simulink model "fir_fft"  (R2022a)
settings: Solver=VariableStepAuto  StartTime=0.0  StopTime=1024*inf  RelTol=1e-3
undefined symbols (not defined in the file): S, taps_td, vsva2197, xcvc1902
libraries: aieBasic x5, aieDSP x2, dspsrcs4 x1, vmcUtilities x1
settings Model: Creator=abehbood  LastModifiedBy=abehbood
settings ModelReferenceCC: EnableRefExpFcnMdlSchedulingChecks=off
settings RTWCC: Description=Generic Real-Time Target

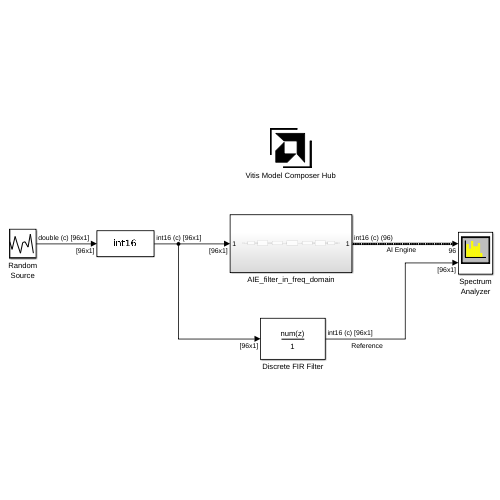
[thumbnail: Simulink's stored preview of the top-level diagram]
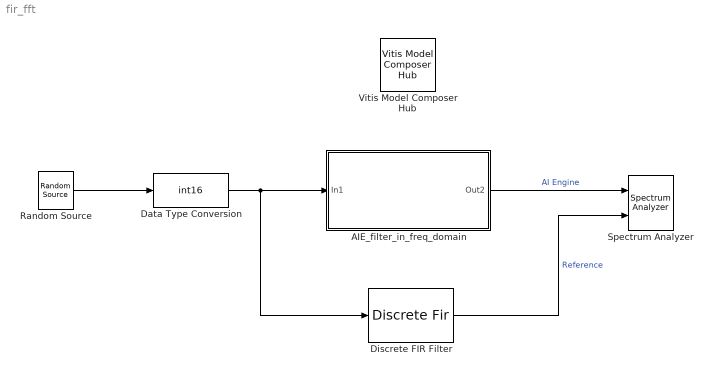
== system fir_fft ==
  AIE_filter_in_freq_domain : Subsystem
  Data Type Conversion : DataTypeConversion  OutDataTypeStr=int16  SaturateOnIntegerOverflow=off  RndMeth=Floor
  Discrete FIR Filter : DiscreteFir  Coefficients=taps_td  InputProcessing=Columns as channels (frame based)  RndMeth=Convergent  SaturateOnIntegerOverflow=on  OutDataTypeStr=Inherit: Same as input
  Random Source : dspsrcs4/Random Source  SrcType=Uniform  NormMethod=Ziggurat  CltLength=12  MinVal=-2^8  MaxVal=2^8  MeanVal=0  VarVal=200  RepMode=Not repeatable  rawSeed=1  IsInherit=off  SampMode=Discrete  SampTime=1  SampFrame=96  DataType=Double  OutComplex=Complex  OutputFrames=off
  Spectrum Analyzer : SpectrumAnalyzer  NumInputPorts=2
  Vitis Model Composer Hub : vmcUtilities/Vitis Model Composer Hub  Tag=genX  CodeGeneration=off  SubsystemName=AIE_filter_in_freq_domain  TargetDirectory=./code  ExportType=AI Engines  IpVendor=xilinx.com  IpLibrary=hls  IpVersion=1.0  IpHWLanguage=Verilog  AieCompilerOptions={}  AieSimulatorOptions={}  CreateTestbench=on  TestbenchStackSize=10  RunAieSim=on  AieSimTimeout=50000  RunAieSimProfiling=off  LaunchVitisAnalyzer=off  PlotOutput=off  RunX86Sim=off  X86SimTimeout=10  GenHwImage=off  PlatformType=Specify Platform  Platform=/proj/xbuilds/SWIP/9999.0_0124_0703/installs/lin64/Vitis/2023.1/base_platforms/xilinx_vck190_base_202310_1/xilinx_vck190_base_202310_1.xpfm  HwSystemType=Baremetal  HwValidationTarget=hw  ProjDevice=xcvc1902-vsva2197-2MP-e-S  ProjDevicePart=xcvc1902-vsva2197-2MP-e-S  SamplePeriod=-1  ClockFrequency=200  DataPathParallelism=1  xilinxfamily=versalaicore  part=xcvc1902  speed=-2MP-e-S  package=vsva2197  directory=./netlist  testbench=off  incr_netlist=off  synthesis_tool=Vivado  clock_wrapper=Clock Enables  dbl_ovrd=According to Block Masks  dcm_input_clock_period=10  sysclk_period=10  simulink_period=1  eval_field=0  LogFileName=''  NThreads=4
  wires:
  Random Source/1 -> Data Type Conversion/1
  Data Type Conversion/1 -> Discrete FIR Filter/1, AIE_filter_in_freq_domain/1(In1)
  Discrete FIR Filter/1 -> Spectrum Analyzer/2  "Reference"
  AIE_filter_in_freq_domain/1(Out2) -> Spectrum Analyzer/1  "AI Engine"

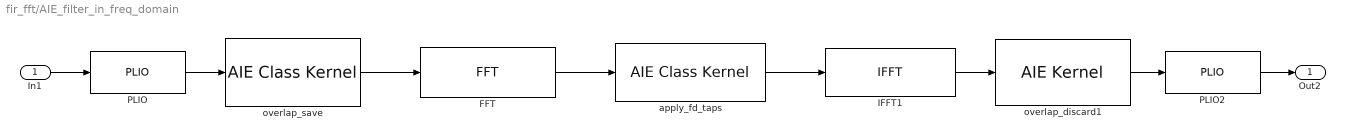
== system fir_fft/AIE_filter_in_freq_domain ==
  In1 : Inport
  FFT : aieDSP/FFT  data_type=cint16  point_size=128  input_window_size=128  shift_val=4  casc_length=1  blockJsonConstraints=[]  blockJsonConstraintsInternal="{\"type\":\"constraint\",\"constraintType\":\"coreUtilization\",\"sid\":\"5:fft_graph.FFTwinproc.m_fftKernels[0]\",\"lhs\":{\"type\":\"runtimeRatio\",\"args\":{\"type\":\"kernel\",\"name\":\"fir_fft/AIE_filter_in_freq_domain/FFT\",\"sid\":\"5:fft_graph.FFTwinproc.m_fftKernels[0]\"}},\"rhs\":{\"type\":\"evaluable\",\"expr\":\"0.9\",\"value\":0.9},\"equality\":true}"  spec=vmc_fft.json  SerializedMaskParamNames=[]  SerializedMaskParamValues=[]  SerializedMaskParamVisibilities=[]
  IFFT1 : aieDSP/IFFT  data_type=cint16  point_size=128  input_window_size=128  shift_val=3  casc_length=1  blockJsonConstraints=[]  blockJsonConstraintsInternal=[]  spec=vmc_ifft.json  SerializedMaskParamNames=[]  SerializedMaskParamValues=[]  SerializedMaskParamVisibilities=[]
  PLIO : aieBasic/PLIO  PlioWidth=64  PlioFreqSpec=off  PlioFreq=250  ColLocation=0  channel=0  blockJsonConstraints=[]  deprecateConstraints=0
  PLIO2 : aieBasic/PLIO  PlioWidth=64  PlioFreqSpec=off  PlioFreq=250  ColLocation=0  channel=0  blockJsonConstraints=[]  deprecateConstraints=0
  apply_fd_taps : aieBasic/AIE Class Kernel  KernelAllAttrs=|  PortNames={'win_i'; 'win_o'}  PortSerializedTypes={'{Q2{R{Tadf::input_buffer{2{t{Scint16}}{t{Tadf::extents{1{t{}128}}}}}}}}'; '{Q2{R{Tadf::output_buffer{2{t{Scint16}}{t{Tadf::extents{1{t{}128}}}}}}}}'}  PortWindowSizes={1.280000000000000000e+02; 1.280000000000000000e+02}  PortWindowMargins={0.000000000000000000e+00; 0.000000000000000000e+00}  PortSynchronicities={'sync', 'sync'}  PortSignalSizes={0.000000000000000000e+00; 0.000000000000000000e+00}  ClassTemplateSpecKind=none  ClassTemplateParamNames={}  ClassTemplateParamKinds={}  ClassTemplateParamTypes={}  ClassTemplateParamValues={}  ClassCtorParamNames={'taps'}  ClassCtorParamSerializedTypes={'{R{Q1{C{Scint16}128}}}'}  ClassCtorParamValues={'[]'}  ClassIndex=1  ClassCtorIndex=1  ClassTabVisible=on  ClassTemplateParamsVisible=off  ClassCtorDeclVisible=on  ClassCtorParamsVisible=on  FunctionTabVisible=on  FunctionDecl=|  PortAttrs={ 'input', 'win_i', 'adf::input_buffer< cint16, adf::extents< 128 > > & restrict', '128', '0', 'sync', ''; 'output', 'win_o', 'adf::output_buffer< cint16, adf::extents< 128 > > & restrict', '128', '', 'sync', '' }  PortAttrsEnables={'off', 'off', 'off', 'off', 'off', 'off', 'off';'off', 'off', 'off', 'off', 'off', 'off', 'off'}  SampleTime=-1  ClassDeclTypeOptions=C[1 1]@t18@class ApplyFdTaps;  ClassDecl=class ApplyFdTaps;  ClassTemplateParams={}  ClassTemplateParamsEnables={}  ClassCtorDeclTypeOptions=C[1 1]@t44@ApplyFdTaps(cint16 const ( & taps ) [ 128 ])  ClassCtorDecl=ApplyFdTaps(cint16 const ( & taps ) [ 128 ])  ClassCtorParams={ 'taps', 'cint16 const ( &) [ 128 ]', 'taps_fd*2^15' }  KernelHeaderFile=kernels/kernels.h  KernelClassName=ApplyFdTaps  KernelFunction=apply_fd_taps  KernelSourceFile=kernels/apply_fd_taps.cpp  KernelSearchPaths={}  PreProcOptions={}  CoreRuntimeRatio=0.9  KernelLocSpec=off  ColRowLocation=[0 0]  blockJsonConstraints=[]  deprecateConstraints=0
      KernelAllAttrs=|
      | s[12;12;9;9;19;14;21;23;21;23;24;21;15;17;12;24;26;26;26;27;28;9;21;23;23;23;24;25;14;19;19;29]@FunctionNameDeclFileNamePortNamesPortTypesPortSerializedTypesPortDirectionsPortWindowSizeEnablesPortWindowMarginEnablesPortBufferSizeEnablesPortBufferMarginEnablesPortSynchronicityEnablesPortSignalSizeEnablesPortBufferSizesPortBufferMarginsFunctionDeclFunctionTemplateSpecKindFunctionTemplateParamNamesFunctionTemplateParamKindsFunctionTemplateParamTypesFunctionTemplateParamValuesFunctionTemplateParamEnablesClassDeclClassTemplateSpecKindClassTemplateParamNamesClassTemplateParamKindsClassTemplateParamTypesClassTemplateParamValuesClassTemplateParamEnablesClassCtorDeclsClassCtorParamNamesClassCtorParamTypesClassCtorParamSerializedTypes[1 1]@C[32 1]@t13@apply_fd_tapst23@../../kernels/kernels.hC[2 1]@t5@win_it5@win_oC[2 1]@t59@adf::input_buffer< cint16, adf::extents< 128 > > & restrictt60@adf::output_buffer< cint16, adf::extents< 128 > > & restrictC[2 1]@t71@{Q2{R{Tadf::input_buffer{2{t{Scint16}}{t{Tadf::extents{1{t{}128}}}}}}}}t72@{Q2{R{Tadf::output_buffer{2{t{Scint16}}{t{Tadf::extents{1{t{}128}}}}}}}}C[2 1]@t5@inputt6@outputC[2 1]@l1@l1@C[2 1]@l1@l0@C[2 1]@l1@l1@C[2 1]@l0@l0@C[2 1]@l1@l1@C[2 1]@l0@l0@C[2 1]@t3@128t3@128C[2 1]@nnt167@void ApplyFdTaps::
      | apply_fd_taps(adf::input_buffer< cint16, adf::extents< 128 > > & restrict win_i, adf::output_buffer< cint16, adf::extents< 128 > > & restrict win_o)t4@nonee[0 1]@e[0 1]@e[0 1]@e[0 1]@e[0 1]@t18@class ApplyFdTaps;t4@nonee[0 1]@e[0 1]@e[0 1]@e[0 1]@e[0 1]@C[1 1]@t44@ApplyFdTaps(cint16 const ( & taps ) [ 128 ])C[1 1]@C[1 1]@t4@tapsC[1 1]@C[1 1]@t25@cint16 const ( &) [ 128 ]C[1 1]@C[1 1]@t22@{R{Q1{C{Scint16}128}}}
      FunctionDecl=|
      | void ApplyFdTaps::
      | apply_fd_taps(adf::input_buffer< cint16, adf::extents< 128 > > & restrict win_i, adf::output_buffer< cint16, adf::extents< 128 > > & restrict win_o)
  overlap_discard1 : aieBasic/AIE Kernel  KernelAllAttrs=s[12;12;9;9;19;14;21;23;21;23;24;21;15;17;12;24;26;26;26;27;28;9;21;23;23;23;24;25;14;19;19;29]@FunctionNameDeclFileNamePortNamesPortTypesPortSerializedTypesPortDirectionsPortWindowSizeEnablesPortWindowMarginEnablesPortBufferSizeEnablesPortBufferMarginEnablesPortSynchronicityEnablesPortSignalSizeEnablesPortBufferSizesPortBufferMarginsFunctionDeclFunctionTemplateSpecKindFunctionTemplateParamNamesFunctionTemplateParamKindsFunctionTemplateParamTypesFunctionTemplateParamValuesFunctionTemplateParamEnablesClassDeclClassTemplateSpecKindClassTemplateParamNamesClassTemplateParamKindsClassTemplateParamTypesClassTemplateParamValuesClassTemplateParamEnablesClassCtorDeclsClassCtorParamNamesClassCtorParamTypesClassCtorParamSerializedTypes[1 1]@C[32 1]@t15@overlap_discardt23@../../kernels/kernels.hC[2 1]@t5@win_it5@win_oC[2 1]@t59@adf::input_buffer< cint16, adf::extents< 128 > > & restrictt59@adf::output_buffer< cint16, adf::extents< 96 > > & restrictC[2 1]@t71@{Q2{R{Tadf::input_buffer{2{t{Scint16}}{t{Tadf::extents{1{t{}128}}}}}}}}t71@{Q2{R{Tadf::output_buffer{2{t{Scint16}}{t{Tadf::extents{1{t{}96}}}}}}}}C[2 1]@t5@inputt6@outputC[2 1]@l1@l1@C[2 1]@l1@l0@C[2 1]@l1@l1@C[2 1]@l0@l0@C[2 1]@l1@l1@C[2 1]@l0@l0@C[2 1]@t3@128t2@96C[2 1]@nnt154@void overlap_discard(adf::input_buffer< cint16, adf::extents< 128 > > & restrict win_i, adf::output_buffer< cint16, adf::extents< 96 > > & restrict win_o)t4@nonee[0 1]@e[0 1]@e[0 1]@e[0 1]@e[0 1]@nne[0 1]@e[0 1]@e[0 1]@e[0 1]@e[0 1]@e[0 1]@e[0 1]@e[0 1]@e[0 1]@  PortNames={'win_i'; 'win_o'}  PortSerializedTypes={'{Q2{R{Tadf::input_buffer{2{t{Scint16}}{t{Tadf::extents{1{t{}128}}}}}}}}'; '{Q2{R{Tadf::output_buffer{2{t{Scint16}}{t{Tadf::extents{1{t{}96}}}}}}}}'}  PortWindowSizes={1.280000000000000000e+02, 9.600000000000000000e+01}  PortWindowMargins={0.000000000000000000e+00, 0.000000000000000000e+00}  PortSynchronicities={'sync', 'sync'}  PortSignalSizes={0.000000000000000000e+00; 0.000000000000000000e+00}  FunctionTemplateSpecKind=none  FunctionTemplateParamNames={}  FunctionTemplateParamKinds={}  FunctionTemplateParamTypes={}  FunctionTemplateParamValues={}  FunctionIndex=1  FunctionTabVisible=on  FunctionTemplateParamsVisible=off  FunctionDeclTypeOptions=C[1 1]@t156@void overlap_discard(adf::input_buffer< cint16, adf::extents< 128 > > && restrict win_i, adf::output_buffer< cint16, adf::extents< 96 > > && restrict win_o)  FunctionDecl=void overlap_discard(adf::input_buffer< cint16, adf::extents< 128 > > && restrict win_i, adf::output_buffer< cint16, adf::extents< 96 > > && restrict win_o)  FunctionTemplateParams={}  FunctionTemplateParamsEnables={}  PortAttrs={ 'input', 'win_i', 'adf::input_buffer< cint16, adf::extents< 128 > > & restrict', '128', '0', 'sync', ''; 'output', 'win_o', 'adf::output_buffer< cint16, adf::extents< 96 > > & restrict', '96', '', 'sync', '' }  PortAttrsEnables={'off', 'off', 'off', 'off', 'off', 'off', 'off';'off', 'off', 'off', 'off', 'off', 'off', 'off'}  SampleTime=-1  KernelHeaderFile=kernels/kernels.h  KernelFunction=overlap_discard  KernelSourceFile=kernels/overlap_discard.cpp  KernelSearchPaths={}  PreProcOptions={}  CoreRuntimeRatio=0.9  KernelLocSpec=off  ColRowLocation=[0 0]  blockJsonConstraints=[]  deprecateConstraints=0
  overlap_save : aieBasic/AIE Class Kernel  KernelAllAttrs=|  PortNames={'win_i'; 'win_o'}  PortSerializedTypes={'{Q2{R{Tadf::input_buffer{2{t{Scint16}}{t{Tadf::extents{1{t{}96}}}}}}}}'; '{Q2{R{Tadf::output_buffer{2{t{Scint16}}{t{Tadf::extents{1{t{}128}}}}}}}}'}  PortWindowSizes={9.600000000000000000e+01; 1.280000000000000000e+02}  PortWindowMargins={0.000000000000000000e+00; 0.000000000000000000e+00}  PortSynchronicities={'sync', 'sync'}  PortSignalSizes={0.000000000000000000e+00; 0.000000000000000000e+00}  ClassTemplateSpecKind=none  ClassTemplateParamNames={}  ClassTemplateParamKinds={}  ClassTemplateParamTypes={}  ClassTemplateParamValues={}  ClassCtorParamNames={}  ClassCtorParamSerializedTypes={}  ClassCtorParamValues={}  ClassIndex=1  ClassCtorIndex=0  ClassTabVisible=on  ClassTemplateParamsVisible=off  ClassCtorDeclVisible=off  ClassCtorParamsVisible=off  FunctionTabVisible=on  FunctionDecl=|  PortAttrs={ 'input', 'win_i', 'adf::input_buffer< cint16, adf::extents< 96 > > & restrict', '96', '0', 'sync', ''; 'output', 'win_o', 'adf::output_buffer< cint16, adf::extents< 128 > > & restrict', '128', '', 'sync', '' }  PortAttrsEnables={'off', 'off', 'off', 'off', 'off', 'off', 'off';'off', 'off', 'off', 'off', 'off', 'off', 'off'}  SampleTime=-1  ClassDeclTypeOptions=C[1 1]@t18@class OverlapSave;  ClassDecl=class OverlapSave;  ClassTemplateParams={}  ClassTemplateParamsEnables={}  ClassCtorDeclTypeOptions=C[1 1]@t7@<empty>  ClassCtorDecl=<empty>  ClassCtorParams={}  KernelHeaderFile=kernels/kernels.h  KernelClassName=OverlapSave  KernelFunction=overlap_save  KernelSourceFile=kernels/overlap_save.cpp  KernelSearchPaths={'./kernels'}  PreProcOptions={}  CoreRuntimeRatio=0.9  KernelLocSpec=off  ColRowLocation=[0 0]  blockJsonConstraints="{\"type\":\"constraint\",\"constraintType\":\"coreUtilization\",\"sid\":\"2\",\"lhs\":{\"type\":\"runtimeRatio\",\"args\":{\"type\":\"kernel\",\"name\":\"fir_fft/AIE_filter_in_freq_domain/overlap_save\",\"sid\":\"2\"}},\"rhs\":{\"type\":\"evaluable\",\"expr\":\"0.1\",\"value\":0.1},\"equality\":true}"  deprecateConstraints=0
      KernelAllAttrs=|
      | s[12;12;9;9;19;14;21;23;21;23;24;21;15;17;12;24;26;26;26;27;28;9;21;23;23;23;24;25;14;19;19;29]@FunctionNameDeclFileNamePortNamesPortTypesPortSerializedTypesPortDirectionsPortWindowSizeEnablesPortWindowMarginEnablesPortBufferSizeEnablesPortBufferMarginEnablesPortSynchronicityEnablesPortSignalSizeEnablesPortBufferSizesPortBufferMarginsFunctionDeclFunctionTemplateSpecKindFunctionTemplateParamNamesFunctionTemplateParamKindsFunctionTemplateParamTypesFunctionTemplateParamValuesFunctionTemplateParamEnablesClassDeclClassTemplateSpecKindClassTemplateParamNamesClassTemplateParamKindsClassTemplateParamTypesClassTemplateParamValuesClassTemplateParamEnablesClassCtorDeclsClassCtorParamNamesClassCtorParamTypesClassCtorParamSerializedTypes[1 1]@C[32 1]@t12@overlap_savet23@../../kernels/kernels.hC[2 1]@t5@win_it5@win_oC[2 1]@t58@adf::input_buffer< cint16, adf::extents< 96 > > & restrictt60@adf::output_buffer< cint16, adf::extents< 128 > > & restrictC[2 1]@t70@{Q2{R{Tadf::input_buffer{2{t{Scint16}}{t{Tadf::extents{1{t{}96}}}}}}}}t72@{Q2{R{Tadf::output_buffer{2{t{Scint16}}{t{Tadf::extents{1{t{}128}}}}}}}}C[2 1]@t5@inputt6@outputC[2 1]@l1@l1@C[2 1]@l1@l0@C[2 1]@l1@l1@C[2 1]@l0@l0@C[2 1]@l1@l1@C[2 1]@l0@l0@C[2 1]@t2@96t3@128C[2 1]@nnt165@void OverlapSave::
      | overlap_save(adf::input_buffer< cint16, adf::extents< 96 > > & restrict win_i, adf::output_buffer< cint16, adf::extents< 128 > > & restrict win_o)t4@nonee[0 1]@e[0 1]@e[0 1]@e[0 1]@e[0 1]@t18@class OverlapSave;t4@nonee[0 1]@e[0 1]@e[0 1]@e[0 1]@e[0 1]@e[0 1]@e[0 1]@e[0 1]@e[0 1]@
      FunctionDecl=|
      | void OverlapSave::
      | overlap_save(adf::input_buffer< cint16, adf::extents< 96 > > & restrict win_i, adf::output_buffer< cint16, adf::extents< 128 > > & restrict win_o)
  Out2 : Outport
  wires:
  overlap_save/1 -> FFT/1
  In1/1 -> PLIO/1
  PLIO/1 -> overlap_save/1
  IFFT1/1 -> overlap_discard1/1
  overlap_discard1/1 -> PLIO2/1
  PLIO2/1 -> Out2/1
  FFT/1 -> apply_fd_taps/1
  apply_fd_taps/1 -> IFFT1/1
